simulink model "Sim_trim"  (R2024b)
settings: Solver=VariableStepAuto  StartTime=0.0  StopTime=10.0  RelTol=1e-3
model workspace (MAT data in the model file):
  VD = 0.8
values from neighbouring files (symbols this model uses):
  A1 = [-(Rg+Ron)/LM	0;  0 -1/(R*C)]    [Matrici_de_stare.m]    (also in PCT_F.m; PCT_F_magda.m; Pct_A_B_C.m; Pct_D_E.m)
  A2 = [-Rg/(LM*(1+n))	  -1/(LM*(1+n));   1/C	-1/(R*C)]    [Matrici_de_stare.m]    (also in PCT_F.m = [-Rg/(LM*(1+ n))	  -1/(LM*(1+n));   1/C	-1/(R*C)]; PCT_F_magda.m = [-Rg/(LM*(1+ n))	  -1/(LM*(1+n));   1/C	-1/(R*C)]; Pct_A_B_C.m; Pct_D_E.m = [-Rg/(LM*(1+ n))	  -1/(LM*(1+n));   1/C	-1/(R*C)])
  B1 = [1/LM 0;  0  0]    [Matrici_de_stare.m]    (also in PCT_F.m; PCT_F_magda.m; Pct_A_B_C.m; Pct_D_E.m)
  B2 = [1/(LM*(1+n)) -1/(LM*(1+n));  0  0]    [Matrici_de_stare.m]    (also in PCT_F.m; PCT_F_magda.m; Pct_A_B_C.m; Pct_D_E.m)
  F1 = [0 0; 0 0]    [Matrici_de_stare.m]    (also in PCT_F.m; PCT_F_magda.m; Pct_A_B_C.m; Pct_D_E.m)
  F2 = [0 0; 0 0]    [Matrici_de_stare.m]    (also in PCT_F.m; PCT_F_magda.m; Pct_A_B_C.m; Pct_D_E.m)
  Vg = 5    [Matrici_de_stare.m]    (also in PCT_F.m; PCT_F_magda.m; Pct_A_B_C.m; Pct_D_E.m)
settings Model: Creator=iorga  LastModifiedBy=iorga

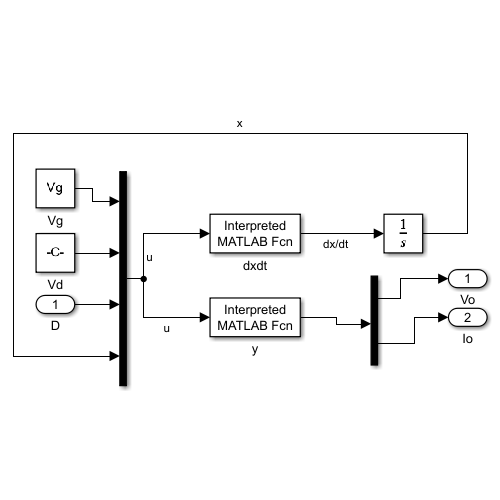
[thumbnail: Simulink's stored preview of the top-level diagram]
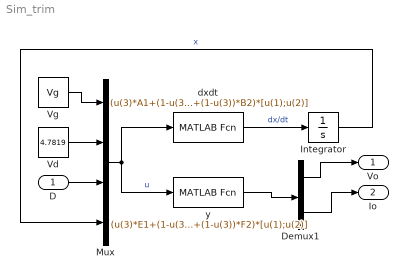
== system Sim_trim ==
  D : Inport
  Demux1 : Demux  Outputs=2
  Integrator : Integrator  InitialCondition=|
      | [3.4161
      |  ;  24.0000]
  Mux : Mux
  Vd : Constant  Value=4.7819
  Vg : Constant  Value=Vg
  dxdt : MATLABFcn  MATLABFcn=(u(3)*A1+(1-u(3))*A2)*[u(4);u(5)]+(u(3)*B1+(1-u(3))*B2)*[u(1);u(2)]  OutputDimensions=2
  y : MATLABFcn  MATLABFcn=(u(3)*E1+(1-u(3))*E2)*[u(4);u(5)]+(u(3)*F1+(1-u(3))*F2)*[u(1);u(2)]  OutputDimensions=2
  Vo : Outport
  Io : Outport  Port=2
  wires:
  Mux/1 -> y/1, dxdt/1  "u"
  Demux1/1 -> Vo/1
  Vg/1 -> Mux/1
  D/1 -> Mux/3
  dxdt/1 -> Integrator/1  "dx/dt"
  y/1 -> Demux1/1
  Integrator/1 -> Mux/4  "x"
  Demux1/2 -> Io/1
  Vd/1 -> Mux/2
